simulink model "Collibration_acceleraiton_brake"  (R2020b)
settings: Solver=VariableStepAuto  StartTime=0.01  StopTime=15  RelTol=1e-3
undefined symbols (not defined in the file): aubr, tablebr, vubr
libraries: Solver_SF x1, pid_lib x1, simulink x1
settings Model: Creator=wwcong  LastModifiedBy=85304
settings DataIOCC: ReturnWorkspaceOutputs=off
settings DebuggingCC: ArithmeticOperatorsInVariantConditions=warning
settings SFSimCC: SimUseLocalCustomCode=off  CustomCodeUndefinedFunction=UseInterfaceOnly
settings RTWCC: RTWUseLocalCustomCode=off

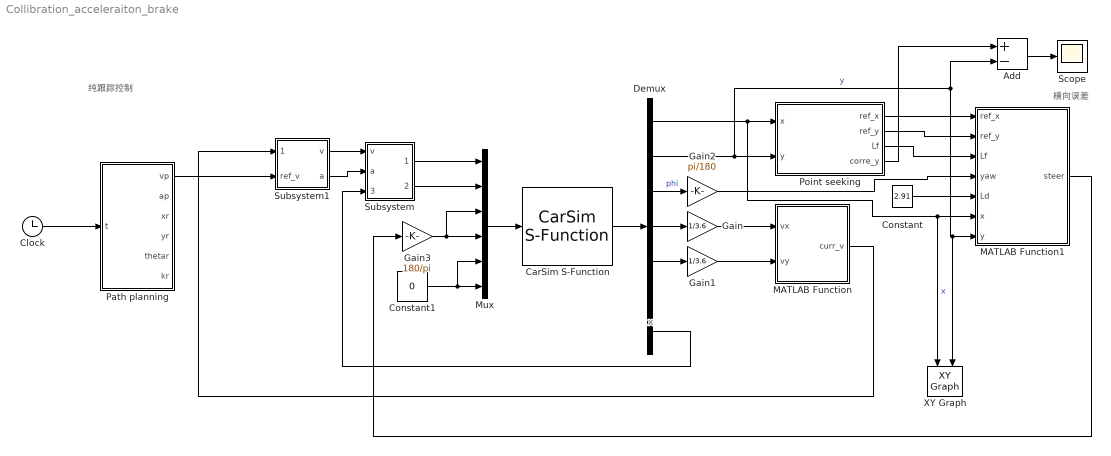
== system Collibration_acceleraiton_brake ==
  note: 横向误差
  note: 纯跟踪控制
  note: x
  Add : Sum  Inputs=+-
  CarSim S-Function : Solver_SF/CarSim S-Function  Priority=1  SIMFILE=Radar_Acc_ExtSen_Car_1.sim
  Clock : Clock
  Constant : Constant  Value=2.91
  Constant1 : Constant  Value=0
  Demux : Demux  Outputs=7
  Gain : Gain  Gain=1/3.6
  Gain1 : Gain  Gain=1/3.6
  Gain2 : Gain  Gain=pi/180
  Gain3 : Gain  Gain=180/pi
  MATLAB Function : MATLAB Function  TreatAsAtomicUnit=on
  MATLAB Function1 : MATLAB Function  TreatAsAtomicUnit=on
  Mux : Mux  Inputs=6
  Path planning : MATLAB Function  TreatAsAtomicUnit=on
  Point seeking : MATLAB Function  TreatAsAtomicUnit=on
  Scope : Scope
  Subsystem : Subsystem
  Subsystem1 : Subsystem
  XY Graph : simulink/Sinks/XY Graph  xmin=0  xmax=80  ymin=0  ymax=20  st=-1
  wires:
  CarSim S-Function/1 -> Demux/1
  Mux/1 -> CarSim S-Function/1
  Subsystem/1(torque) -> Mux/1
  Subsystem/2(brake) -> Mux/2
  Subsystem1/1(v) -> Subsystem/1(v)
  Demux/4 -> Gain/1
  Demux/5 -> Gain1/1
  Demux/7 -> Subsystem/3(rpm)
  Gain/1 -> MATLAB Function/1(vx)
  Gain1/1 -> MATLAB Function/2(vy)
  MATLAB Function/1(curr_v) -> Subsystem1/1(current_v)
  Clock/1 -> Path planning/1(t)
  Demux/1 -> MATLAB Function1/6(x), XY Graph/1, Point seeking/1(x)  "x"
  Demux/2 -> Add/2, MATLAB Function1/7(y), XY Graph/2, Point seeking/2(y)  "y"
  Demux/3 -> Gain2/1  "phi"
  Point seeking/1(ref_x) -> MATLAB Function1/1(ref_x)
  Point seeking/2(ref_y) -> MATLAB Function1/2(ref_y)
  Gain2/1 -> MATLAB Function1/4(yaw)
  Constant/1 -> MATLAB Function1/5(Ld)
  Point seeking/3(Lf) -> MATLAB Function1/3(Lf)
  Constant1/1 -> Mux/5, Mux/6
  Gain3/1 -> Mux/4, Mux/3
  MATLAB Function1/1(steer) -> Gain3/1
  Path planning/1(vp) -> Subsystem1/2(ref_v)
  Add/1 -> Scope/1
  Point seeking/4(corre_y) -> Add/1
  Subsystem1/2(a) -> Subsystem/2(a)

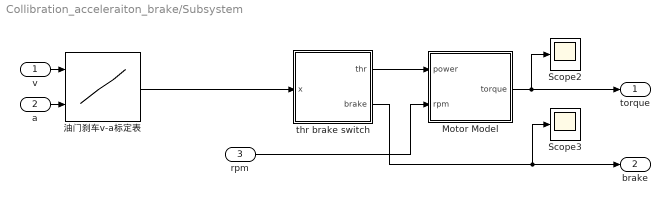
== system Collibration_acceleraiton_brake/Subsystem ==
  v : Inport
  a : Inport  Port=2
  rpm : Inport  Port=3
  Motor Model : MATLAB Function  TreatAsAtomicUnit=on
  Scope2 : Scope
  Scope3 : Scope
  thr brake switch : MATLAB Function  TreatAsAtomicUnit=on
  油门刹车v-a标定表 : Lookup_n-D  BreakpointsForDimension1=vubr  BreakpointsForDimension2=aubr  Table=tablebr  InternalRulePriority=Speed  RndMeth=Simplest  InputSameDT=on
      settings: InputPortMap=u0,u1
  torque : Outport
  brake : Outport  Port=2
  wires:
  v/1 -> 油门刹车v-a标定表/1
  thr brake switch/2(brake) -> brake/1, Scope3/1
  rpm/1 -> Motor Model/2(rpm)
  thr brake switch/1(thr) -> Motor Model/1(power)
  a/1 -> 油门刹车v-a标定表/2
  Motor Model/1(torque) -> torque/1, Scope2/1
  油门刹车v-a标定表/1 -> thr brake switch/1(x)

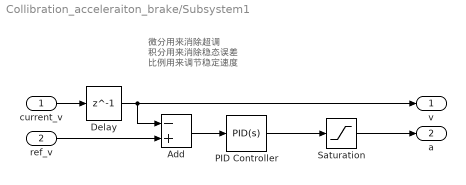
== system Collibration_acceleraiton_brake/Subsystem1 ==
  note: 微分用来消除超调
      | 积分用来消除稳态误差
      | 比例用来调节稳定速度
  current_v : Inport
  ref_v : Inport  Port=2
  Add : Sum  Inputs=-+
  Delay : Delay  DelayLength=1
  PID Controller : pid_lib/PID Controller  Controller=PID  Form=Parallel  TimeDomain=Continuous-time  UseExternalTs=off  SampleTime=-1  IntegratorMethod=Forward Euler  FilterMethod=Forward Euler  ControllerParametersSource=internal  P=1  I=0  D=0.1  UseFilter=on  N=30  TunerSelectOption=Transfer Function Based (PID Tuner App)  InitialConditionSource=internal  InitialConditionForIntegrator=0  InitialConditionForFilter=0  DifferentiatorICPrevScaledInput=0  ExternalReset=none  TrackingMode=off  Kt=1  LimitOutput=off  SatLimitsSource=internal  UpperSaturationLimit=inf  LowerSaturationLimit=-inf  LinearizeAsGain=on  AntiWindupMode=none  Kb=1  POutMin=[]  POutMax=[]  IOutMin=[]  IOutMax=[]  DOutMin=[]  DOutMax=[]  NOutMin=[]  NOutMax=[]  SumOutMin=[]  SumOutMax=[]  SaturationOutMin=[]  SaturationOutMax=[]  PParamMin=[]  PParamMax=[]  IParamMin=[]  IParamMax=[]  DParamMin=[]  DParamMax=[]  NParamMin=[]  NParamMax=[]  KbParamMin=[]  KbParamMax=[]  KtParamMin=[]  KtParamMax=[]  KbOutMin=[]  KbOutMax=[]  KtOutMin=[]  KtOutMax=[]  IntegratorOutMin=[]  IntegratorOutMax=[]  FilterOutMin=[]  FilterOutMax=[]  SumI1OutMin=[]  SumI1OutMax=[]  SumI2OutMin=[]  SumI2OutMax=[]  SumI3OutMin=[]  SumI3OutMax=[]  SumI4OutMin=[]  SumI4OutMax=[]  SumDOutMin=[]  SumDOutMax=[]  DifferentiatorOutMin=[]  DifferentiatorOutMax=[]  FilterDiffOutCoefMin=[]  FilterDiffOutCoefMax=[]  ReciprocalOutMin=[]  ReciprocalOutMax=[]  SumDenOutMin=[]  SumDenOutMax=[]  SumNumOutMin=[]  SumNumOutMax=[]  DivideOutMin=[]  DivideOutMax=[]  UdiffTsProdOutMin=[]  UdiffTsProdOutMax=[]  NTsProdOutMin=[]  NTsProdOutMax=[]  UintegralTsProdOutMin=[]  UintegralTsProdOutMax=[]  UngainTsProdOutMin=[]  UngainTsProdOutMax=[]  IntegratorContinuousStateAttributes=''  IntegratorStateMustResolveToSignalObject=off  IntegratorRTWStateStorageClass=Auto  FilterContinuousStateAttributes=''  FilterStateMustResolveToSignalObject=off  FilterRTWStateStorageClass=Auto  ParallelPVariant=InternalParameters  IdealPVariant=Disabled  IVariant=InternalParameters  DVariant=InternalParameters  IntegratorVariant=Continuous  SatVariant=Disabled  AWVariant=Passthrough  PCopyVariant=Disabled  TRVariant=Disabled  FdbkBlocksVariant=Forward  IdealPFdbkVariant=Disabled  SatFdbkVariant=Disabled  DerivativeFilterVariant=ContFilter  NVariant=InternalParameters  NCopyVariant=Disabled  FilterICVariant=InternalICsFilter  IntegratorICVariant=InternalICs  ExternalResetVariant=Disabled  TRSumVariant=Passthrough  SumFdbkVariant=Disabled  SumVariant=Sum_PID  TsampFilterVariant=InternalTs  TsampNgainVariant=Passthrough  TsampIntegralVariant=Passthrough  ExternalSaturationOutDataTypeStr=Inherit: Same as second input
  Saturation : Saturate  UpperLimit=5  LowerLimit=-8
  v : Outport
  a : Outport  Port=2
  wires:
  Delay/1 -> v/1, Add/1
  Add/1 -> PID Controller/1
  PID Controller/1 -> Saturation/1
  Saturation/1 -> a/1
  current_v/1 -> Delay/1
  ref_v/1 -> Add/2

== matlab function Collibration_acceleraiton_brake/Subsystem/thr brake switch ==
  data: x input; thr output; brake output
function [thr,brake] = trans(x)

    if(x>0)
        thr=x;
        brake=0;
    else 
        thr=0;
        brake=-x;
    end
end

== matlab function Collibration_acceleraiton_brake/Subsystem/Motor Model ==
  data: power input; torque output; rpm input
function torque = fcn(power,rpm)
Tmax=400*power;
    if(rpm<=4523)
        torque=Tmax;
    else 
        torque=Tmax*4523/rpm;
    end
end

== matlab function Collibration_acceleraiton_brake/MATLAB Function ==
  data: vx input; curr_v output; vy input
function curr_v = fcn(vx,vy)
curr_v=sqrt(vx^2+vy^2);

== matlab function Collibration_acceleraiton_brake/MATLAB Function1 ==
  data: ref_x input; steer output; ref_y input; Lf input; yaw input; Ld input; x input; y input
function steer = fcn(ref_x,ref_y,Lf,yaw,Ld,x,y)

alpha=atan2(ref_y-y,ref_x-x)-yaw; % atan2函数计算点（x,y）与x轴正向夹角,即atan2(y,x).
steer=atan2(2.0*Ld*sin(alpha)/Lf,1.0);

== matlab function Collibration_acceleraiton_brake/Point seeking ==
  data: x input; ref_x output; y input; ref_y output; Lf output; corre_y output
function [ref_x,ref_y,Lf,corre_y] = seek(x,y)
xo=50;
yo=5;
A=[1   0   0   0   0   0;                       % 求解五次多项式系数
   0   1   0   0   0   0;
   0   0   2   0   0   0;
   1   xo  xo^2  xo^3 xo^4  xo^5;
   0   1  2*xo 3*xo^2 4*xo^3 5*xo^4;
   0   0   2   6*xo 12*xo^2 20*xo^3];
B=[0;0;0;yo;0;0];
X5=linsolve(A,B);
x1=0:0.01:xo;
y1=X5(1)+X5(2).*x1+X5(3)*x1.^2+X5(4)*x1.^3+X5(5).*x1.^4+X5(6).*x1.^5;

idx=0;
LL=1; % 预瞄距离
i=length(y1(1,:));
 while(1)            
  
            D=norm([x-x1(1,i) y-y1(1,i)]);  % 计算两个点之间的直线距离函数
            i=i-1;
            if(i<1)
                i=1;
                break;
            end
            if(D<=LL)
                idx=i;
                break;
            end
 end
 
 ref_x=x1(idx);
 ref_y=y1(idx);
 Lf=LL;
 
 corre_y=X5(1)+X5(2)*x+X5(3)*x^2+X5(4)*x^3+X5(5)*x^4+X5(6)*x^5;

== matlab function Collibration_acceleraiton_brake/Path planning ==
  data: t input; vp output; ap output; xr output; yr output; thetar output; kr output
function [vp,ap,xr,yr,thetar,kr] = fcn(t)
    dx=50;
    dy=5;
    T=8;
    xstart=[0,0,0];
    xend=[dx,0,0];
    ystart=[0,0,0];
    yend=[dy,0,0];
    a=zeros(1,6);
    b=zeros(1,6);
    
    a(1)=xstart(1);
    a(2)=xstart(2);
    a(3)=xstart(3)/2;
    A1=[T^3,T^4,T^5;
        3*T^2,4*T^3,5*T^4;
        6*T,12*T^2,20*T^3];
    B1=[xend(1)-a(1)-a(2)*T-a(3)*T^2;
        xend(2)-a(2)-2*a(3)*T;
        xend(3)-2*a(3)];
    xs=inv(A1)*B1;
    a(4)=xs(1);
    a(5)=xs(2);
    a(6)=xs(3);
    b(1)=ystart(1);
    b(2)=ystart(2);
    b(3)=ystart(3)/2;
    A2=[dx^3,dx^4,dx^5;
        3*dx^2,4*dx^3,5*dx^4;
        6*dx,12*dx^2,20*dx^3];
    B2=[yend(1)-b(1)-b(2)*dx-b(3)*dx^2;
        yend(2)-b(2)-2*b(3)*dx;
        yend(3)-2*b(3)];
    ys=inv(A2)*B2;
    b(4)=ys(1);
    b(5)=ys(2);
    b(6)=ys(3);
    xr=a(1)+a(2)*t+a(3)*t^2+a(4)*t^3+a(5)*t^4+a(6)*t^5;
    yr=b(1)+b(2)*xr+b(3)*xr^2+b(4)*xr^3+b(5)*xr^4+b(6)*xr^5;
    xr_dot=a(2)+2*a(3)*t+3*a(4)*t^2+4*a(5)*t^3+5*a(6)*t^4;
    yr_dx=b(2)+2*b(3)*xr+3*b(4)*xr^2+4*b(5)*xr^3+5*b(6)*xr^4;
    yr_dot=yr_dx*xr_dot;
    thetar=atan(yr_dx);
    xr_dot2=2*a(3)+6*a(4)*t+12*a(5)*t^2+20*a(6)*t^3;
    yr_dx2=2*b(3)+6*b(4)*xr+12*b(5)*xr^2+20*b(6)*xr^3;
    yr_dot2=yr_dx2*xr_dot^2+yr_dx*xr_dot2;
    kr=yr_dx2/((1+yr_dx^2)^1.5);
    vp=sqrt(xr_dot^2+yr_dot^2);
    if xr_dot2>=0
        ap=sqrt(xr_dot2^2+yr_dot2^2);
    else
        ap=-sqrt(xr_dot2^2+yr_dot2^2);
    end
